simulink model "PT_model"  (R2022a)
settings: Solver=VariableStepAuto  StartTime=0.0  StopTime=inf  RelTol=1e-3
values from neighbouring files (symbols this model uses):
  a = 1    [ev_mod1.m]    (also in ev_model.m)
  ap = 1.07    [ev_mod1.m]    (also in ev_model.m)
  ce = 0.9    [ev_mod1.m]    (also in ev_model.m)
  cell_c = 5    [ev_mod1.m]    (also in ev_model.m)
  cell_v = 3.6    [ev_mod1.m]    (also in ev_model.m)
  gr = 9.81    [ev_mod1.m]    (also in ev_model.m = 9.2)
  lap = 17    [ev_mod1.m]    (also in ev_model.m = 10)
  me = 0.85    [ev_mod1.m]    (also in ev_model.m)
  ocv = data(:,2)    [ev_mod1.m]    (also in ev_model.m)
  rho = 1.225    [ev_mod1.m]    (also in ev_model.m)
  rw = 0.2921    [ev_mod1.m]    (also in ev_model.m)
  soc = data(:,1)    [ev_mod1.m]    (also in ev_model.m)
  te = 0.78    [ev_mod1.m]    (also in ev_model.m = 0.88)
  v = 48    [ev_mod1.m]    (also in ev_model.m)
settings Model: SimulationMode=accelerator  Creator=Sai Vivek  LastModifiedBy=Sai Vivek

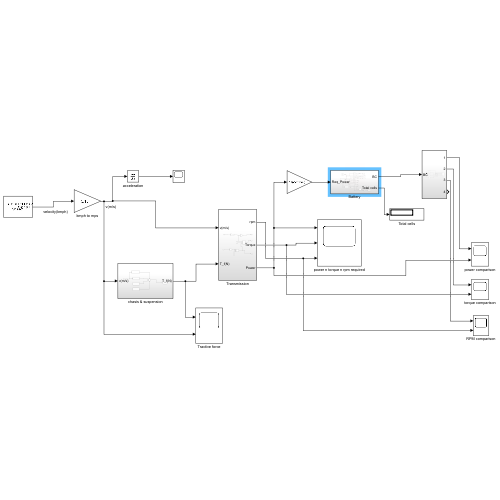
[thumbnail: Simulink's stored preview of the top-level diagram]
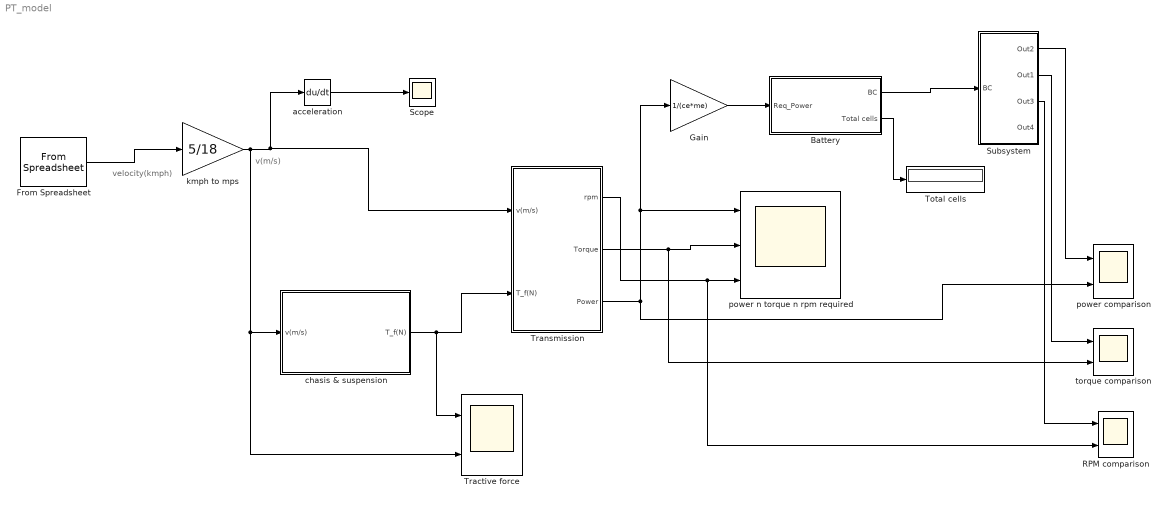
== system PT_model ==
  note: velocity(kmph)
  note: v(m/s)
  Battery : Subsystem
  From Spreadsheet : FromSpreadsheet  FileName=SUPPLY EDITED BY2.xlsx  Range=A1:B601
  Gain : Gain  Gain=1/(ce*me)
  RPM comparison : Scope  NumInputPorts=2
  Scope : Scope
  Subsystem : Subsystem
  Total cells : Display
  Tractive force : Scope  NumInputPorts=2
  Transmission : Subsystem
  acceleration : Derivative
  chasis & suspension : Subsystem
  kmph to mps : Gain  Gain=5/18
  power comparison : Scope  NumInputPorts=2
  power n torque n rpm required : Scope  NumInputPorts=3
  torque comparison : Scope  NumInputPorts=2
  wires:
  From Spreadsheet/1 -> kmph to mps/1
  kmph to mps/1 -> Transmission/1(v(m/s)), acceleration/1, Tractive force/2, chasis & suspension/1(v(m/s))
  acceleration/1 -> Scope/1
  Transmission/3(Power) -> power n torque n rpm required/1, Gain/1, power comparison/2
  Gain/1 -> Battery/1(Req_Power)
  Battery/2(Total cells) -> Total cells/1
  Battery/1(BC) -> Subsystem/1(BC)
  Subsystem/1(Out2) -> power comparison/1
  Subsystem/2(Out1) -> torque comparison/1
  Subsystem/3(Out3) -> RPM comparison/1
  Transmission/2(Torque) -> torque comparison/2, power n torque n rpm required/2
  Transmission/1(rpm) -> RPM comparison/2, power n torque n rpm required/3
  chasis & suspension/1(T_f(N)) -> Tractive force/1, Transmission/2(T_f(N))

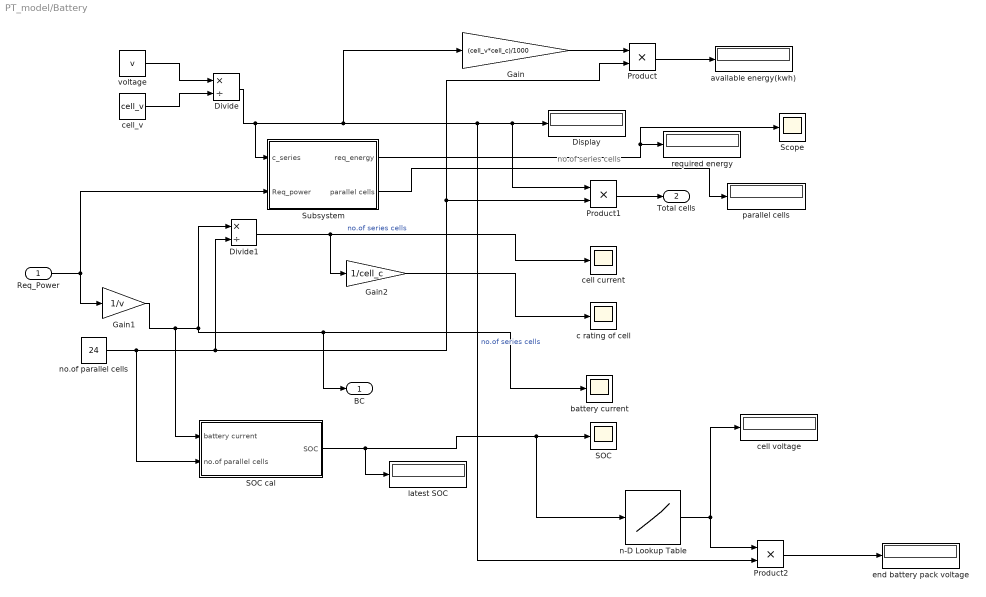
== system PT_model/Battery ==
  note: no.of series cells
  Req_Power : Inport
  Display : Display
  Divide : Product  Inputs=*/
  Divide1 : Product  Inputs=*/
  Gain : Gain  Gain=(cell_v*cell_c)/1000
  Gain1 : Gain  Gain=1/v
  Gain2 : Gain  Gain=1/cell_c
  Product : Product
  Product1 : Product
  Product2 : Product
  SOC : Scope
  SOC cal : Subsystem
  Scope : Scope
  Subsystem : Subsystem
  available energy(kwh) : Display
  battery current : Scope
  c rating of cell : Scope
  cell current : Scope
  cell voltage : Display
  cell_v : Constant  Value=cell_v
  end battery pack voltage : Display
  latest SOC : Display
  n-D Lookup Table : Lookup_n-D  NumberOfTableDimensions=1  BreakpointsForDimension1=soc  BreakpointsForDimension3=[5, 7]  Table=ocv  InternalRulePriority=Speed  RndMeth=Simplest
  no.of parallel cells : Constant  Value=24
  parallel cells : Display
  required energy : Display
  voltage : Constant  Value=v
  BC : Outport
  Total cells : Outport  Port=2
  wires:
  voltage/1 -> Divide/1
  cell_v/1 -> Divide/2
  Divide/1 -> Subsystem/1(c_series), Gain/1, Product2/2, Product1/1, Display/1  "no.of series cells"
  Gain/1 -> Product/1
  no.of parallel cells/1 -> SOC cal/2(no.of parallel cells), Divide1/2, Product1/2, Product/2
  Product/1 -> available energy(kwh)/1
  Product1/1 -> Total cells/1
  Req_Power/1 -> Subsystem/2(Req_power), Gain1/1
  Gain1/1 -> SOC cal/1(battery current), Divide1/1, BC/1, battery current/1
  Divide1/1 -> Gain2/1, cell current/1  "no.of series cells"
  Gain2/1 -> c rating of cell/1
  SOC cal/1(SOC) -> latest SOC/1, n-D Lookup Table/1, SOC/1
  n-D Lookup Table/1 -> cell voltage/1, Product2/1
  Product2/1 -> end battery pack voltage/1
  Subsystem/1(req_energy) -> Scope/1, required energy/1
  Subsystem/2(parallel cells) -> parallel cells/1

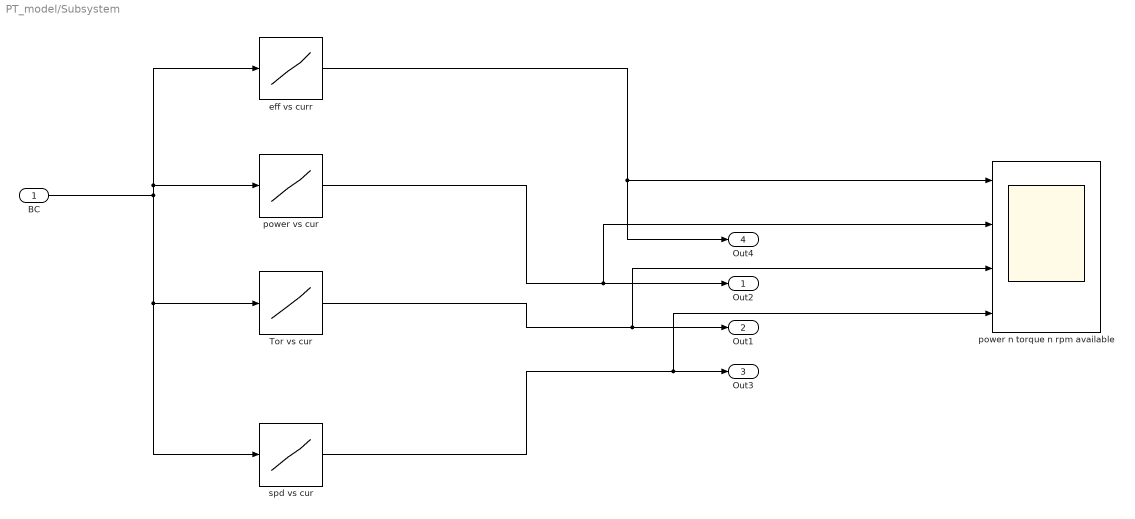
== system PT_model/Subsystem ==
  BC : Inport
  Tor vs cur : Lookup_n-D  NumberOfTableDimensions=1  BreakpointsForDimension1=soc  BreakpointsForDimension3=[5, 7]  Table=ocv  InternalRulePriority=Speed  RndMeth=Simplest
  eff vs curr : Lookup_n-D  NumberOfTableDimensions=1  BreakpointsForDimension1=soc  BreakpointsForDimension3=[5, 7]  Table=ocv  InternalRulePriority=Speed  RndMeth=Simplest
  power n torque n rpm available : Scope  NumInputPorts=4
  power vs cur : Lookup_n-D  NumberOfTableDimensions=1  BreakpointsForDimension1=soc  BreakpointsForDimension3=[5, 7]  Table=ocv  InternalRulePriority=Speed  RndMeth=Simplest
  spd vs cur : Lookup_n-D  NumberOfTableDimensions=1  BreakpointsForDimension1=soc  BreakpointsForDimension3=[5, 7]  Table=ocv  InternalRulePriority=Speed  RndMeth=Simplest
  Out2 : Outport
  Out1 : Outport  Port=2
  Out3 : Outport  Port=3
  Out4 : Outport  Port=4
  wires:
  BC/1 -> power vs cur/1, eff vs curr/1, spd vs cur/1, Tor vs cur/1
  power vs cur/1 -> power n torque n rpm available/2, Out2/1
  Tor vs cur/1 -> power n torque n rpm available/3, Out1/1
  spd vs cur/1 -> power n torque n rpm available/4, Out3/1
  eff vs curr/1 -> power n torque n rpm available/1, Out4/1

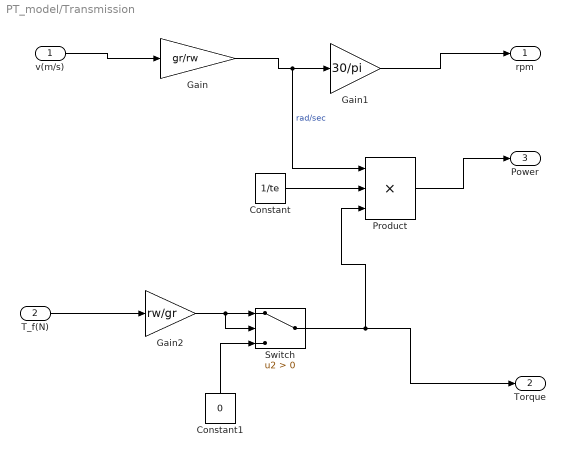
== system PT_model/Transmission ==
  v(m/s) : Inport
  T_f(N) : Inport  Port=2
  Constant : Constant  Value=1/te
  Constant1 : Constant  Value=0
  Gain : Gain  Gain=gr/rw
  Gain1 : Gain  Gain=30/pi
  Gain2 : Gain  Gain=rw/gr
  Product : Product  Inputs=3
  Switch : Switch  Criteria=u2 > Threshold  SaturateOnIntegerOverflow=off  InputSameDT=off
  rpm : Outport
  Torque : Outport  Port=2
  Power : Outport  Port=3
  wires:
  v(m/s)/1 -> Gain/1
  Gain/1 -> Product/1, Gain1/1  "rad/sec"
  Gain1/1 -> rpm/1
  T_f(N)/1 -> Gain2/1
  Constant/1 -> Product/2
  Product/1 -> Power/1
  Switch/1 -> Product/3, Torque/1
  Gain2/1 -> Switch/1, Switch/2
  Constant1/1 -> Switch/3

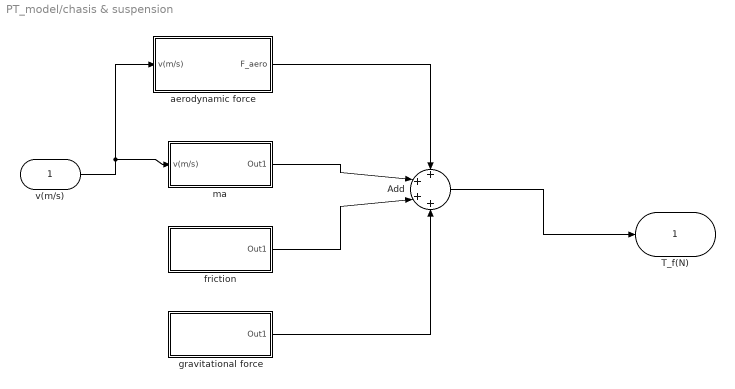
== system PT_model/chasis & suspension ==
  v(m/s) : Inport
  Add : Sum  Inputs=++++
  aerodynamic force : Subsystem
  friction : Subsystem
  gravitational force : Subsystem
  ma : Subsystem
  T_f(N) : Outport
  wires:
  v(m/s)/1 -> ma/1(v(m/s)), aerodynamic force/1(v(m/s))
  aerodynamic force/1(F_aero) -> Add/1
  ma/1(Out1) -> Add/2
  friction/1(Out1) -> Add/3
  gravitational force/1(Out1) -> Add/4
  Add/1 -> T_f(N)/1

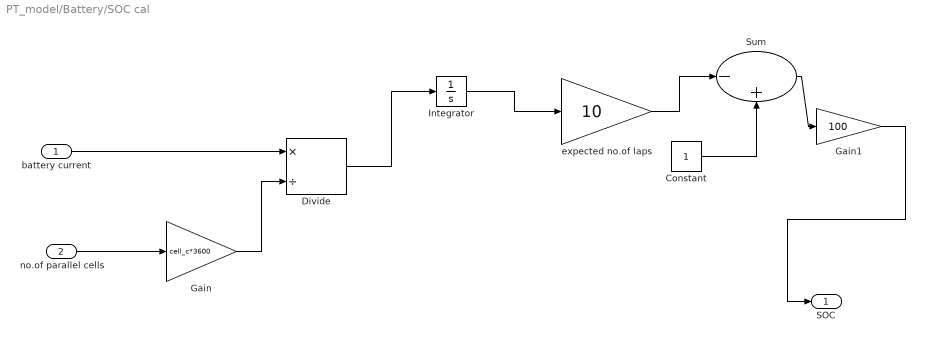
== system PT_model/Battery/SOC cal ==
  battery current : Inport
  no.of parallel cells : Inport  Port=2
  Constant : Constant
  Divide : Product  Inputs=*/
  Gain : Gain  Gain=cell_c*3600
  Gain1 : Gain  Gain=100
  Integrator : Integrator
  Sum : Sum  Inputs=|-+
  expected no.of laps : Gain  Gain=10
  SOC : Outport
  wires:
  no.of parallel cells/1 -> Gain/1
  Gain/1 -> Divide/2
  battery current/1 -> Divide/1
  Divide/1 -> Integrator/1
  Integrator/1 -> expected no.of laps/1
  expected no.of laps/1 -> Sum/1
  Constant/1 -> Sum/2
  Sum/1 -> Gain1/1
  Gain1/1 -> SOC/1

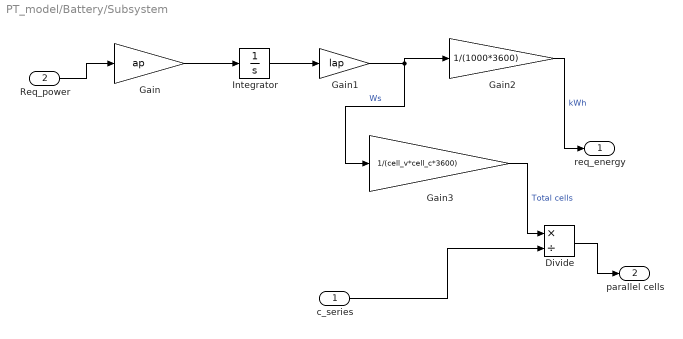
== system PT_model/Battery/Subsystem ==
  c_series : Inport
  Req_power : Inport  Port=2
  Divide : Product  Inputs=*/
  Gain : Gain  Gain=ap
  Gain1 : Gain  Gain=lap
  Gain2 : Gain  Gain=1/(1000*3600)
  Gain3 : Gain  Gain=1/(cell_v*cell_c*3600)
  Integrator : Integrator
  req_energy : Outport
  parallel cells : Outport  Port=2
  wires:
  Req_power/1 -> Gain/1
  Gain/1 -> Integrator/1
  Integrator/1 -> Gain1/1
  Gain1/1 -> Gain3/1, Gain2/1  "Ws"
  Gain2/1 -> req_energy/1  "kWh"
  Gain3/1 -> Divide/1  "Total cells"
  c_series/1 -> Divide/2
  Divide/1 -> parallel cells/1

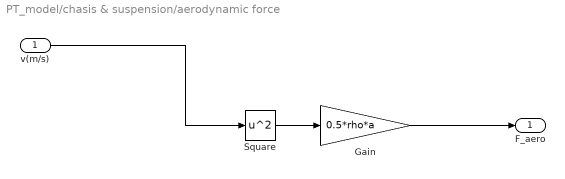
== system PT_model/chasis & suspension/aerodynamic force ==
  v(m/s) : Inport
  Gain : Gain  Gain=0.5*rho*a
  Square : Math  Operator=square
  F_aero : Outport
  wires:
  v(m/s)/1 -> Square/1
  Square/1 -> Gain/1
  Gain/1 -> F_aero/1

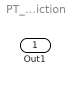
== system PT_model/chasis & suspension/friction ==
  Out1 : Outport
  wires:
  ? -> Out1/1

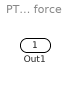
== system PT_model/chasis & suspension/gravitational force ==
  Out1 : Outport
  wires:
  ? -> Out1/1

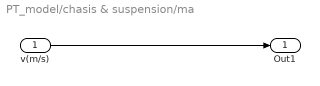
== system PT_model/chasis & suspension/ma ==
  v(m/s) : Inport
  Out1 : Outport
  wires:
  v(m/s)/1 -> Out1/1
